simulink model "TST_BusCreatorForwardOptimization"  (Simulink 7.4)
settings: Solver=FixedStepDiscrete  StartTime=0.0  StopTime=10.0  FixedStep=0.02  RelTol=1e-3
settings Model: Creator=kharthforeign  LastModifiedBy=kharthforeign  BufferReuse=off
settings DataIOCC: SaveOutput=off  SignalLogging=off  SaveTime=off
settings OptimizationCC: BlockReduction=off  ConditionallyExecuteInputs=off  OptimizeBlockIOStorage=off  BufferReuse=off  ExpressionFolding=off  LocalBlockOutputs=off  InitFltsAndDblsToZero=on

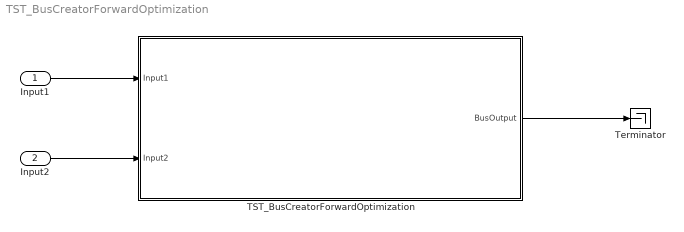
== system TST_BusCreatorForwardOptimization ==
  Input1 : Inport  DataType=double  OutDataType=fixdt(1, 16)  OutScaling=2^0  OutDataTypeStr=double  BusOutputAsStruct=on
  Input2 : Inport  Port=2  PortDimensions=1  DataType=uint32  OutDataType=fixdt(1, 16)  OutScaling=2^0  OutDataTypeStr=uint32  BusOutputAsStruct=on
  TST_BusCreatorForwardOptimization : Subsystem  TreatAsAtomicUnit=on
  Terminator : Terminator
  wires:
  Input1/1 -> TST_BusCreatorForwardOptimization/1(Input1)
  Input2/1 -> TST_BusCreatorForwardOptimization/2(Input2)
  TST_BusCreatorForwardOptimization/1(BusOutput) -> Terminator/1

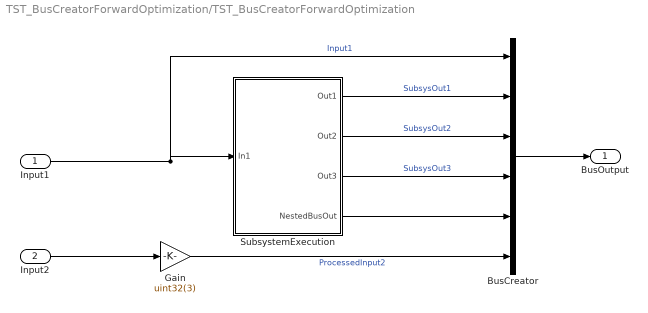
== system TST_BusCreatorForwardOptimization/TST_BusCreatorForwardOptimization ==
  Input1 : Inport  PortDimensions=1  DataType=double  OutDataType=fixdt(1, 16)  OutScaling=2^0  OutDataTypeStr=double  BusOutputAsStruct=on
  Input2 : Inport  Port=2  PortDimensions=1  DataType=uint32  OutDataType=fixdt(1, 16)  OutScaling=2^0  OutDataTypeStr=uint32  BusOutputAsStruct=on
  BusCreator : BusCreator  Inputs=6  NonVirtualBus=on
  Gain : Gain  Gain=uint32(3)  ParameterDataTypeMode=uint32  ParameterDataType=fixdt(1, 16)  ParameterScaling=2^0  ParamDataTypeStr=uint32  OutDataTypeMode=uint32  OutDataType=fixdt(1, 16)  OutScaling=2^0  OutDataTypeStr=uint32
  SubsystemExecution : Subsystem  TreatAsAtomicUnit=on
  BusOutput : Outport  OutDataType=fixdt(1, 16)  OutScaling=2^0  BusOutputAsStruct=on
  wires:
  BusCreator/1 -> BusOutput/1
  Input1/1 -> SubsystemExecution/1(In1), BusCreator/1  "Input1"
  Input2/1 -> Gain/1
  SubsystemExecution/1(Out1) -> BusCreator/2  "SubsysOut1"
  SubsystemExecution/2(Out2) -> BusCreator/3  "SubsysOut2"
  SubsystemExecution/3(Out3) -> BusCreator/4  "SubsysOut3"
  Gain/1 -> BusCreator/6  "ProcessedInput2"
  SubsystemExecution/4(NestedBusOut) -> BusCreator/5

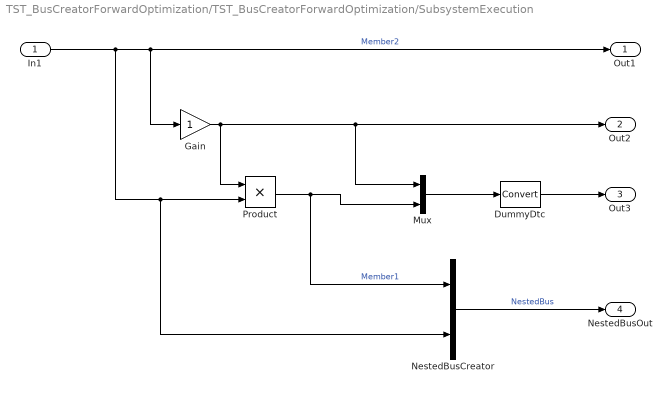
== system TST_BusCreatorForwardOptimization/TST_BusCreatorForwardOptimization/SubsystemExecution ==
  In1 : Inport  OutDataType=fixdt(1, 16)  OutScaling=2^0
  DummyDtc : DataTypeConversion  OutDataType=fixdt(1, 16)  OutScaling=2^0
  Gain : Gain  ParameterDataType=fixdt(1, 16)  ParameterScaling=2^0  OutDataType=fixdt(1, 16)  OutScaling=2^0
  Mux : Mux  Inputs=2
  NestedBusCreator : BusCreator  Inputs=2  NonVirtualBus=on
  Product : Product  OutDataType=fixdt(1, 16)  OutScaling=2^0  RndMeth=Zero
  Out1 : Outport  OutDataType=fixdt(1, 16)  OutScaling=2^0
  Out2 : Outport  Port=2  OutDataType=fixdt(1, 16)  OutScaling=2^0
  Out3 : Outport  Port=3  OutDataType=fixdt(1, 16)  OutScaling=2^0
  NestedBusOut : Outport  Port=4  OutDataType=fixdt(1, 16)  OutScaling=2^0  BusOutputAsStruct=on
  wires:
  In1/1 -> Out1/1, Gain/1, Product/2, NestedBusCreator/2  "Member2"
  Gain/1 -> Product/1, Out2/1, Mux/1
  Mux/1 -> DummyDtc/1
  Product/1 -> Mux/2, NestedBusCreator/1  "Member1"
  DummyDtc/1 -> Out3/1
  NestedBusCreator/1 -> NestedBusOut/1  "NestedBus"
